simulink model "motorsim"  (R2015b)
settings: Solver=ode4  StartTime=0.0  StopTime=10  FixedStep=0.001  RelTol=1e-3
values from neighbouring files (symbols this model uses):
  alpha = 1/K(1)    [lsrl.m]
  tau = alpha*K(2)    [lsrl.m]
settings Model: ExtModeTrigDuration=10000  Creator=millerid  LastModifiedBy=flynng
settings SolverCC: PositivePriorityOrder=on
settings RTWCC: SystemTargetFile=quarc_win64.tlc  TemplateMakefile=quarc_default_tmf  Description=QUARC Win64 Target
settings STFCustomTargetCC: TargetPreCompLibLocation=C:\ProgramData\QUARC\lib\2015b\win64\release  GeneratePreprocessorConditionals=Use local settings  MatFileLogging=on  CPPClassGenCompliant=off
settings GRTTargetCC: TargetPreCompLibLocation=C:\ProgramData\QUARC\lib\2015b\win64\release  ParMdlRefBuildCompliant=off  CompOptLevelCompliant=off  CombineOutputUpdateFcns=off  CPPClassGenCompliant=off  GRTInterface=on  UseToolchainInfoCompliant=off  ExtMode=on  ExtModeMexFile=quarc_comm

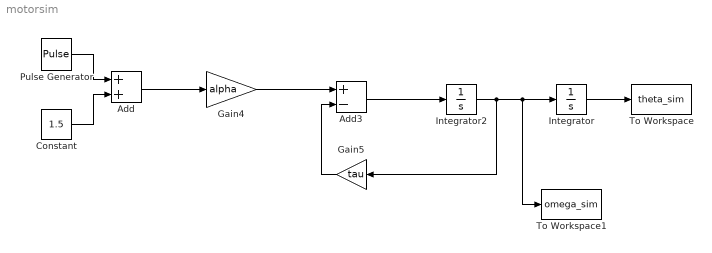
== system motorsim ==
  Add : Sum
  Add3 : Sum  Inputs=+-
  Constant : Constant  Value=1.5
  Gain4 : Gain  Gain=alpha
  Gain5 : Gain  Gain=tau
  Integrator : Integrator
  Integrator2 : Integrator
  Pulse Generator : DiscretePulseGenerator  PulseType=Time based  Amplitude=2  Period=2.5  PulseWidth=50
  To Workspace : ToWorkspace  VariableName=theta_sim  SampleTime=-1
  To Workspace1 : ToWorkspace  VariableName=omega_sim  SampleTime=-1
  wires:
  Constant/1 -> Add/2
  Pulse Generator/1 -> Add/1
  Add/1 -> Gain4/1
  Gain4/1 -> Add3/1
  Gain5/1 -> Add3/2
  Add3/1 -> Integrator2/1
  Integrator2/1 -> To Workspace1/1, Integrator/1, Gain5/1
  Integrator/1 -> To Workspace/1
